simulink model "strelkowa_rep3_FLtransk"  (R2013a)
settings: Solver=ode4  StartTime=0.0  StopTime=3000.0  FixedStep=0.1  RelTol=1e-3
values from neighbouring files (symbols this model uses):
  c2 = 0.12    [evaluation_FL.m]    (also in init_Strelkowa_FLTransk.m)
  c3 = 2.6    [evaluation_FL.m]    (also in init_Strelkowa_FLTransk.m)
  c4 = 0.06    [evaluation_FL.m]    (also in init_Strelkowa_FLTransk.m)
  mRNA_init = 10    [evaluation_FL.m]    (also in init_Strelkowa_FLTransk.m)
libraries: fuzblock x3
settings Model: Creator=Jure Bordon  LastModifiedBy=Jure Bordon
settings DataIOCC: InspectSignalLogs=on

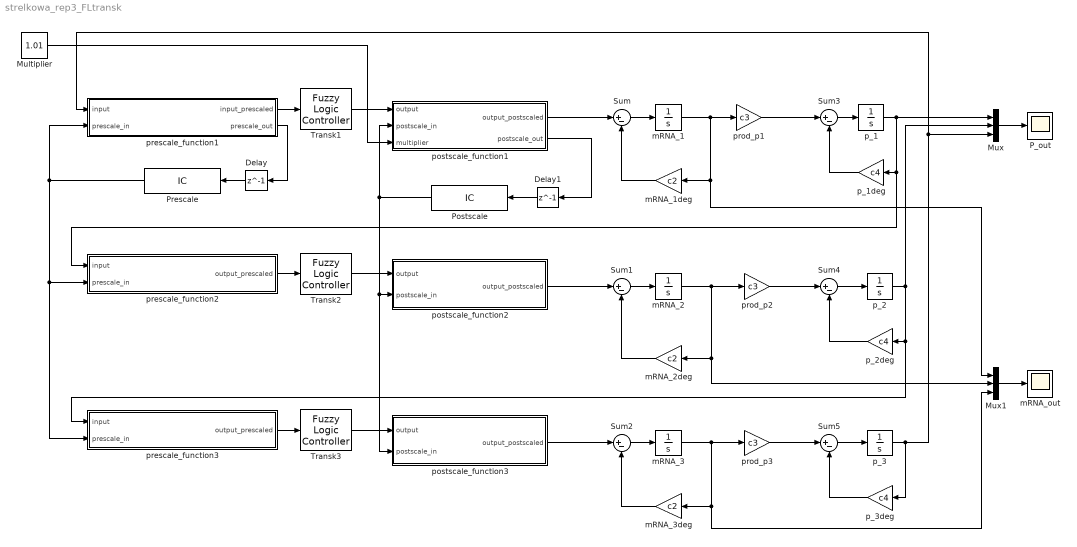
== system strelkowa_rep3_FLtransk ==
  Delay : Delay  DelayLength=1  InitialCondition=1
  Delay1 : Delay  DelayLength=1  InitialCondition=1
  Multiplier : Constant  Value=1.01
  Mux : Mux  Inputs=3
  Mux1 : Mux  Inputs=3
  P_out : Scope
      settings: YMin=0  YMax=1800  SaveName=P_out
  Postscale : InitialCondition
  Prescale : InitialCondition
  Sum{,1..5} (6 alike) : Sum  Inputs=|+-
  Transk1 : fuzblock/Fuzzy Logic  Controller  fis=Transk
  Transk2 : fuzblock/Fuzzy Logic  Controller  fis=Transk
  Transk3 : fuzblock/Fuzzy Logic  Controller  fis=Transk
  mRNA_1 : Integrator  InitialCondition=mRNA_init + 0.5  LimitOutput=on  LowerSaturationLimit=0
  mRNA_1deg : Gain  Gain=c2
  mRNA_2 : Integrator  InitialCondition=mRNA_init  LimitOutput=on  LowerSaturationLimit=0
  mRNA_2deg : Gain  Gain=c2
  mRNA_3 : Integrator  InitialCondition=mRNA_init  LimitOutput=on  LowerSaturationLimit=0
  mRNA_3deg : Gain  Gain=c2
  mRNA_out : Scope
      settings: SaveName=mRNA_out
  p_1 : Integrator  LimitOutput=on  LowerSaturationLimit=0
  p_1deg : Gain  Gain=c4
  p_2 : Integrator  LimitOutput=on  LowerSaturationLimit=0
  p_2deg : Gain  Gain=c4
  p_3 : Integrator  LimitOutput=on  LowerSaturationLimit=0
  p_3deg : Gain  Gain=c4
  postscale_function1 : MATLAB Function  TreatAsAtomicUnit=on
  postscale_function2 : MATLAB Function  TreatAsAtomicUnit=on
  postscale_function3 : MATLAB Function  TreatAsAtomicUnit=on
  prescale_function1 : MATLAB Function  TreatAsAtomicUnit=on
  prescale_function2 : MATLAB Function  TreatAsAtomicUnit=on
  prescale_function3 : MATLAB Function  TreatAsAtomicUnit=on
  prod_p1 : Gain  Gain=c3
  prod_p2 : Gain  Gain=c3
  prod_p3 : Gain  Gain=c3
  wires:
  Sum/1 -> mRNA_1/1
  Sum1/1 -> mRNA_2/1
  Sum2/1 -> mRNA_3/1
  Sum3/1 -> p_1/1
  p_1/1 -> Mux/1, prescale_function2/1(input), p_1deg/1
  p_1deg/1 -> Sum3/2
  Sum4/1 -> p_2/1
  p_2/1 -> p_2deg/1, prescale_function3/1(input), Mux/2
  p_2deg/1 -> Sum4/2
  Sum5/1 -> p_3/1
  p_3/1 -> p_3deg/1, Mux/3, prescale_function1/1(input)
  p_3deg/1 -> Sum5/2
  postscale_function3/1(output_postscaled) -> Sum2/1
  postscale_function2/1(output_postscaled) -> Sum1/1
  Mux/1 -> P_out/1
  mRNA_1/1 -> prod_p1/1, mRNA_1deg/1, Mux1/1
  mRNA_2/1 -> prod_p2/1, mRNA_2deg/1, Mux1/2
  mRNA_3/1 -> mRNA_3deg/1, Mux1/3, prod_p3/1
  Mux1/1 -> mRNA_out/1
  mRNA_1deg/1 -> Sum/2
  mRNA_2deg/1 -> Sum1/2
  mRNA_3deg/1 -> Sum2/2
  prod_p1/1 -> Sum3/1
  prod_p3/1 -> Sum5/1
  prod_p2/1 -> Sum4/1
  prescale_function1/1(input_prescaled) -> Transk1/1
  prescale_function1/2(prescale_out) -> Delay/1
  prescale_function2/1(output_prescaled) -> Transk2/1
  prescale_function3/1(output_prescaled) -> Transk3/1
  Prescale/1 -> prescale_function3/2(prescale_in), prescale_function2/2(prescale_in), prescale_function1/2(prescale_in)
  Transk1/1 -> postscale_function1/1(output)
  Multiplier/1 -> postscale_function1/3(multiplier)
  Transk2/1 -> postscale_function2/1(output)
  Postscale/1 -> postscale_function3/2(postscale_in), postscale_function2/2(postscale_in), postscale_function1/2(postscale_in)
  Transk3/1 -> postscale_function3/1(output)
  postscale_function1/1(output_postscaled) -> Sum/1
  postscale_function1/2(postscale_out) -> Delay1/1
  Delay/1 -> Prescale/1
  Delay1/1 -> Postscale/1

== matlab function strelkowa_rep3_FLtransk/prescale_function2 ==
  data: input input; output_prescaled output; prescale_in input
function output_prescaled  = prescale(input, prescale_in)

output_prescaled = input/prescale_in;

== matlab function strelkowa_rep3_FLtransk/prescale_function1 ==
  data: input input; input_prescaled output; prescale_in input; prescale_out output
function [input_prescaled, prescale_out] = prescale(input, prescale_in)

prescale_out = prescale_in;

if (input > prescale_in)
    prescale_out = input;
end

input_prescaled = input/prescale_out;

== matlab function strelkowa_rep3_FLtransk/prescale_function3 ==
  data: input input; output_prescaled output; prescale_in input
function output_prescaled  = prescale(input, prescale_in)

output_prescaled = input/prescale_in;

== matlab function strelkowa_rep3_FLtransk/postscale_function1 ==
  data: output input; output_postscaled output; postscale_in input; postscale_out output; multiplier input
function [output_postscaled, postscale_out] = postscale(output, postscale_in, multiplier)

postscale_out = postscale_in;

if (output*multiplier > postscale_out)
    postscale_out = output*multiplier;
end

output_postscaled = output*postscale_out;

== matlab function strelkowa_rep3_FLtransk/postscale_function2 ==
  data: output input; output_postscaled output; postscale_in input
function output_postscaled  = postscale(output, postscale_in)
%#codegen

output_postscaled = output*postscale_in;

== matlab function strelkowa_rep3_FLtransk/postscale_function3 ==
  data: output input; output_postscaled output; postscale_in input
function output_postscaled  = postscale(output, postscale_in)

output_postscaled = output*postscale_in;
